simulink model "DOF4_v5"  (R2018a)
settings: Solver=VariableStepAuto  StartTime=0.0  StopTime=20  RelTol=1e-3
undefined symbols (not defined in the file or in its folder): X, Y, Z
libraries: sm_lib x20, nesl_utility x12, simulink x5
settings Model: Creator=sty  LastModifiedBy=sty

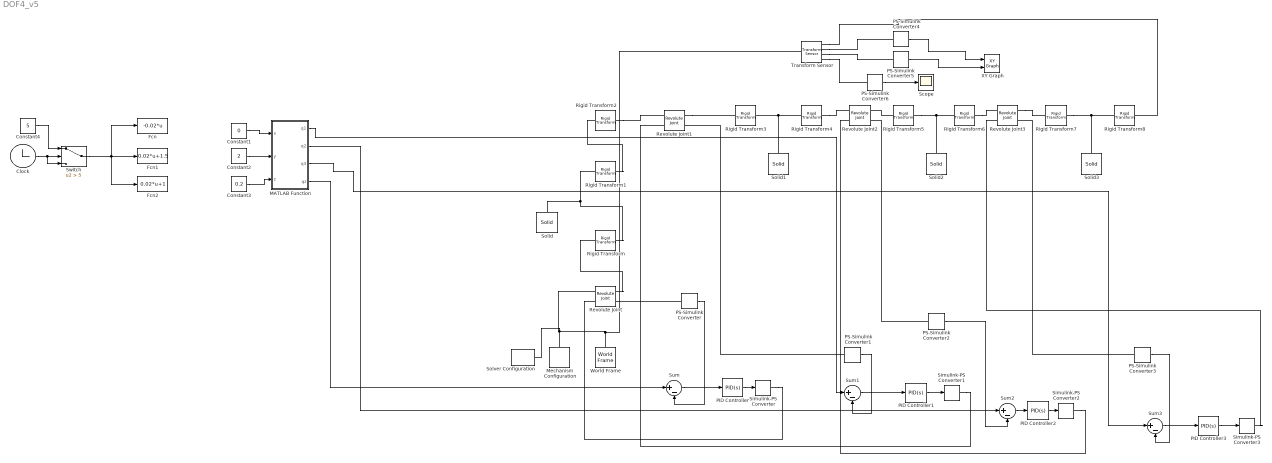
== system DOF4_v5 ==
  Clock : Clock
  Constant1 : Constant  Value=0
  Constant2 : Constant  Value=2
  Constant3 : Constant  Value=0.2
  Constant4 : Constant  Value=5
  Fcn : Fcn  Expr=-0.02*u
  Fcn1 : Fcn  Expr=0.02*u+1.5
  Fcn2 : Fcn  Expr=0.02*u+1
  MATLAB Function : MATLAB Function  TreatAsAtomicUnit=on
  Mechanism Configuration : sm_lib/Utilities/Mechanism Configuration  UniformGravity=Constant  GravityVector=[0 0 0]  GravityUnits=m/s^2  LinearizationDelta=0.001
  PID Controller{,1..3} (4 alike) : simulink/Continuous/PID Controller  Controller=PID  TimeDomain=Continuous-time  SampleTime=-1  IntegratorMethod=Forward Euler  FilterMethod=Forward Euler  Form=Parallel  UseFilter=on  ControllerParametersSource=internal  P=1000  I=40  D=60  N=100  InitialConditionSource=internal  InitialConditionForIntegrator=0  InitialConditionForFilter=0  ExternalReset=none  LimitOutput=off  UpperSaturationLimit=inf  LowerSaturationLimit=-inf  LinearizeAsGain=on  AntiWindupMode=none  Kb=1  TrackingMode=off  Kt=1  PParamMin=[]  PParamMax=[]  IParamMin=[]  IParamMax=[]  DParamMin=[]  DParamMax=[]  NParamMin=[]  NParamMax=[]  KbParamMin=[]  KbParamMax=[]  KtParamMin=[]  KtParamMax=[]  POutMin=[]  POutMax=[]  IOutMin=[]  IOutMax=[]  DOutMin=[]  DOutMax=[]  NOutMin=[]  NOutMax=[]  KbOutMin=[]  KbOutMax=[]  KtOutMin=[]  KtOutMax=[]  IntegratorOutMin=[]  IntegratorOutMax=[]  FilterOutMin=[]  FilterOutMax=[]  SumOutMin=[]  SumOutMax=[]  SumI1OutMin=[]  SumI1OutMax=[]  SumI2OutMin=[]  SumI2OutMax=[]  SumI3OutMin=[]  SumI3OutMax=[]  SumDOutMin=[]  SumDOutMax=[]  SaturationOutMin=[]  SaturationOutMax=[]  IntegratorContinuousStateAttributes=''  IntegratorStateMustResolveToSignalObject=off  IntegratorRTWStateStorageClass=Auto  FilterContinuousStateAttributes=''  FilterStateMustResolveToSignalObject=off  FilterRTWStateStorageClass=Auto  DifferentiatorICPrevScaledInput=0  DifferentiatorOutMin=[]  DifferentiatorOutMax=[]  FilterDiffOutCoefMin=[]  FilterDiffOutCoefMax=[]  SumDenOutMin=[]  SumDenOutMax=[]  SumNumOutMin=[]  SumNumOutMax=[]  ReciprocalOutMin=[]  ReciprocalOutMax=[]  DivideOutMin=[]  DivideOutMax=[]  TunerSelectOption=Transfer Function Based (PID Tuner App)
  PS-Simulink Converter{,1..6} (7 alike) : nesl_utility/PS-Simulink Converter  PhysicalDomain=network_engine_domain  SubClassName=ps_output  LeftPortType=input  RightPortType=output  PseudoPeriodic=off  Frequencies=[]  Unit=1  AffineConversion=off
  Revolute Joint{,1..3} (4 alike) : sm_lib/Joints/Revolute Joint  SenseConstraintForce=off  SenseConstraintForceX=off  SenseConstraintForceY=off  SenseConstraintForceZ=off  SenseConstraintTorque=off  SenseConstraintTorqueX=off  SenseConstraintTorqueY=off  SenseConstraintTorqueZ=off  SenseTotalForce=off  SenseTotalForceX=off  SenseTotalForceY=off  SenseTotalForceZ=off  SenseTotalTorque=off  SenseTotalTorqueX=off  SenseTotalTorqueY=off  SenseTotalTorqueZ=off  CompositeWrenchDir=FollowerOnBase  CompositeWrenchFrame=BaseFrame  EquilibriumPosition=0  EquilibriumPositionUnits=deg  SpringStiffness=0  SpringStiffnessUnits=N*m/deg  DampingCoefficient=0  DampingCoefficientUnits=N*m/(deg/s)  TorqueActuationMode=InputTorque  MotionActuationMode=ComputedMotion  SensePosition=on  SenseVelocity=off  SenseAcceleration=off  SenseTorqueForce=off  PositionTargetSpecify=off  PositionTargetPriority=High  PositionTargetValue=0  PositionTargetValueUnits=deg  VelocityTargetSpecify=off  VelocityTargetPriority=High  VelocityTargetValue=0  VelocityTargetValueUnits=deg/s
  Rigid Transform : sm_lib/Frames and Transforms/Rigid Transform  TranslationMethod=StandardAxis  TranslationStandardOffset=0.1  TranslationLengthUnit=m  TranslationStandardAxis=+Z  TranslationCartesianOffset=[0 0 0]  TranslationROffset=0  TranslationROffsetUnits=m  TranslationZOffset=0  TranslationZOffsetUnits=m  TranslationThetaOffset=0  TranslationThetaOffsetUnits=deg  RotationMethod=None  RotationAngleUnits=deg  RotationStandardAxis=+Z  RotationAngle=0.0  RotationArbitraryAxis=[0 0 1]  FollAlignAxisA=+X  BaseAlignAxisA=+Y  FollAlignAxisB=+Y  BaseAlignAxisB=+Z  RotationSequenceAxes=FollowerAxes  RotationSequence=XYX  RotationSequenceAngles=[0 0 0]  RotationSequenceAnglesUnits=deg  RotationMatrix=[1 0 0; 0 1 0; 0 0 1]
  Rigid Transform1 : sm_lib/Frames and Transforms/Rigid Transform  TranslationMethod=StandardAxis  TranslationStandardOffset=0.1  TranslationLengthUnit=m  TranslationStandardAxis=+Z  TranslationCartesianOffset=[0 0 0]  TranslationROffset=0  TranslationROffsetUnits=m  TranslationZOffset=0  TranslationZOffsetUnits=m  TranslationThetaOffset=0  TranslationThetaOffsetUnits=deg  RotationMethod=None  RotationAngleUnits=deg  RotationStandardAxis=+Z  RotationAngle=0.0  RotationArbitraryAxis=[0 0 1]  FollAlignAxisA=+X  BaseAlignAxisA=+Y  FollAlignAxisB=+Y  BaseAlignAxisB=+Z  RotationSequenceAxes=FollowerAxes  RotationSequence=XYX  RotationSequenceAngles=[0 0 0]  RotationSequenceAnglesUnits=deg  RotationMatrix=[1 0 0; 0 1 0; 0 0 1]
  Rigid Transform2 : sm_lib/Frames and Transforms/Rigid Transform  TranslationMethod=None  TranslationStandardOffset=0.1  TranslationLengthUnit=m  TranslationStandardAxis=+Z  TranslationCartesianOffset=[0 0 0]  TranslationROffset=0  TranslationROffsetUnits=m  TranslationZOffset=0  TranslationZOffsetUnits=m  TranslationThetaOffset=0  TranslationThetaOffsetUnits=deg  RotationMethod=StandardAxis  RotationAngleUnits=deg  RotationStandardAxis=+Y  RotationAngle=-90  RotationArbitraryAxis=[0 0 1]  FollAlignAxisA=+X  BaseAlignAxisA=+Y  FollAlignAxisB=+Y  BaseAlignAxisB=+Z  RotationSequenceAxes=FollowerAxes  RotationSequence=XYX  RotationSequenceAngles=[0 0 0]  RotationSequenceAnglesUnits=deg  RotationMatrix=[1 0 0; 0 1 0; 0 0 1]
  Rigid Transform{3..6} (4 alike) : sm_lib/Frames and Transforms/Rigid Transform  TranslationMethod=StandardAxis  TranslationStandardOffset=0.5  TranslationLengthUnit=m  TranslationStandardAxis=+Y  TranslationCartesianOffset=[0 0 0]  TranslationROffset=0  TranslationROffsetUnits=m  TranslationZOffset=0  TranslationZOffsetUnits=m  TranslationThetaOffset=0  TranslationThetaOffsetUnits=deg  RotationMethod=None  RotationAngleUnits=deg  RotationStandardAxis=+Z  RotationAngle=0.0  RotationArbitraryAxis=[0 0 1]  FollAlignAxisA=+X  BaseAlignAxisA=+Y  FollAlignAxisB=+Y  BaseAlignAxisB=+Z  RotationSequenceAxes=FollowerAxes  RotationSequence=XYX  RotationSequenceAngles=[0 0 0]  RotationSequenceAnglesUnits=deg  RotationMatrix=[1 0 0; 0 1 0; 0 0 1]
  Rigid Transform7 : sm_lib/Frames and Transforms/Rigid Transform  TranslationMethod=StandardAxis  TranslationStandardOffset=0.25  TranslationLengthUnit=m  TranslationStandardAxis=+Y  TranslationCartesianOffset=[0 0 0]  TranslationROffset=0  TranslationROffsetUnits=m  TranslationZOffset=0  TranslationZOffsetUnits=m  TranslationThetaOffset=0  TranslationThetaOffsetUnits=deg  RotationMethod=None  RotationAngleUnits=deg  RotationStandardAxis=+Z  RotationAngle=0.0  RotationArbitraryAxis=[0 0 1]  FollAlignAxisA=+X  BaseAlignAxisA=+Y  FollAlignAxisB=+Y  BaseAlignAxisB=+Z  RotationSequenceAxes=FollowerAxes  RotationSequence=XYX  RotationSequenceAngles=[0 0 0]  RotationSequenceAnglesUnits=deg  RotationMatrix=[1 0 0; 0 1 0; 0 0 1]
  Rigid Transform8 : sm_lib/Frames and Transforms/Rigid Transform  TranslationMethod=StandardAxis  TranslationStandardOffset=0.25  TranslationLengthUnit=m  TranslationStandardAxis=+Y  TranslationCartesianOffset=[0 0 0]  TranslationROffset=0  TranslationROffsetUnits=m  TranslationZOffset=0  TranslationZOffsetUnits=m  TranslationThetaOffset=0  TranslationThetaOffsetUnits=deg  RotationMethod=None  RotationAngleUnits=deg  RotationStandardAxis=+Z  RotationAngle=0.0  RotationArbitraryAxis=[0 0 1]  FollAlignAxisA=+X  BaseAlignAxisA=+Y  FollAlignAxisB=+Y  BaseAlignAxisB=+Z  RotationSequenceAxes=FollowerAxes  RotationSequence=XYX  RotationSequenceAngles=[0 0 0]  RotationSequenceAnglesUnits=deg  RotationMatrix=[1 0 0; 0 1 0; 0 0 1]
  Scope : Scope
  Simulink-PS Converter{,1..3} (4 alike) : nesl_utility/Simulink-PS Converter  PhysicalDomain=network_engine_domain  SubClassName=ps_input  LeftPortType=input  RightPortType=output  PseudoPeriodic=off  Frequencies=[]  NoiseDistribution=none  NoiseParameters=[]  Unit=1  AffineConversion=off  FilteringAndDerivatives=provide  SimscapeFilterOrder=1  InputFilterTimeConstant=0.001  UdotUserProvided=0
  Solid : sm_lib/Body Elements/Solid  InertiaType=CalculateFromGeometry  Mass=1  MassUnits=kg  CenterOfMass=[0 0 0]  CenterOfMassUnits=m  MomentsOfInertia=[1 1 1]  MomentsOfInertiaUnits=kg*m^2  ProductsOfInertia=[0 0 0]  ProductsOfInertiaUnits=kg*m^2  DensityBased=on  Density=1000  DensityUnits=kg/m^3  DoExposeReferenceFrame=on  SerializedFrames=<Frames/>  GraphicType=FromGeometry  MarkerShape=Sphere  MarkerSize=10  GraphicVisPropType=SimpleVisualProperties  GraphicDiffuseColor=[0.0 0.0 1.0]  GraphicSpecularColor=[0.5 0.5 0.5 1.0]  GraphicAmbientColor=[0.15 0.15 0.15 1.0]  GraphicEmissiveColor=[0.0 0.0 0.0 1.0]  GraphicShininess=75  GraphicOpacity=1.0  GeometryShape=Brick  RectangleSize=[1 1]  RectangleSizeUnits=m  BrickDimensions=[0.1 0.1 0.2]  BrickDimensionUnits=m  CylinderRadius=1  CylinderRadiusUnits=m  CylinderLength=1  CylinderLengthUnits=m  SphereRadius=1  SphereRadiusUnits=m  EllipsoidRadii=[1 1 1]  EllipsoidRadiiUnits=m  ExtrusionCrossSection=[1 1; -1 1; -1 -1; 1 -1]  ExtrusionCrossSectionUnits=m  ExtrusionLength=1  ExtrusionLengthUnits=m  PolygonNumSides=3  PolygonOuterRadius=1  PolygonOuterRadiusUnits=m  ExtGeomFileType=STEP  ExtGeomFileUnits=m  RevolutionCrossSection=[1 1; 1 -1; 2 -1; 2 1]  RevolutionCrossSectionUnits=m  RevolutionExtent=Full  RevolutionAngle=180  RevolutionAngleUnits=deg
  Solid1 : sm_lib/Body Elements/Solid  InertiaType=CalculateFromGeometry  Mass=1  MassUnits=kg  CenterOfMass=[0 0 0]  CenterOfMassUnits=m  MomentsOfInertia=[1 1 1]  MomentsOfInertiaUnits=kg*m^2  ProductsOfInertia=[0 0 0]  ProductsOfInertiaUnits=kg*m^2  DensityBased=on  Density=1000  DensityUnits=kg/m^3  DoExposeReferenceFrame=on  SerializedFrames=<Frames/>  GraphicType=FromGeometry  MarkerShape=Sphere  MarkerSize=10  GraphicVisPropType=SimpleVisualProperties  GraphicDiffuseColor=[1.0 1.0 0.2]  GraphicSpecularColor=[0.5 0.5 0.5 1.0]  GraphicAmbientColor=[0.15 0.15 0.15 1.0]  GraphicEmissiveColor=[0.0 0.0 0.0 1.0]  GraphicShininess=75  GraphicOpacity=1.0  GeometryShape=Brick  RectangleSize=[1 1]  RectangleSizeUnits=m  BrickDimensions=[0.1 1 0.1]  BrickDimensionUnits=m  CylinderRadius=1  CylinderRadiusUnits=m  CylinderLength=1  CylinderLengthUnits=m  SphereRadius=1  SphereRadiusUnits=m  EllipsoidRadii=[1 1 1]  EllipsoidRadiiUnits=m  ExtrusionCrossSection=[1 1; -1 1; -1 -1; 1 -1]  ExtrusionCrossSectionUnits=m  ExtrusionLength=1  ExtrusionLengthUnits=m  PolygonNumSides=3  PolygonOuterRadius=1  PolygonOuterRadiusUnits=m  ExtGeomFileType=STEP  ExtGeomFileUnits=m  RevolutionCrossSection=[1 1; 1 -1; 2 -1; 2 1]  RevolutionCrossSectionUnits=m  RevolutionExtent=Full  RevolutionAngle=180  RevolutionAngleUnits=deg
  Solid2 : sm_lib/Body Elements/Solid  InertiaType=CalculateFromGeometry  Mass=1  MassUnits=kg  CenterOfMass=[0 0 0]  CenterOfMassUnits=m  MomentsOfInertia=[1 1 1]  MomentsOfInertiaUnits=kg*m^2  ProductsOfInertia=[0 0 0]  ProductsOfInertiaUnits=kg*m^2  DensityBased=on  Density=1000  DensityUnits=kg/m^3  DoExposeReferenceFrame=on  SerializedFrames=<Frames/>  GraphicType=FromGeometry  MarkerShape=Sphere  MarkerSize=10  GraphicVisPropType=SimpleVisualProperties  GraphicDiffuseColor=[0.0 0.0 1.0]  GraphicSpecularColor=[0.5 0.5 0.5 1.0]  GraphicAmbientColor=[0.15 0.15 0.15 1.0]  GraphicEmissiveColor=[0.0 0.0 0.0 1.0]  GraphicShininess=75  GraphicOpacity=1.0  GeometryShape=Brick  RectangleSize=[1 1]  RectangleSizeUnits=m  BrickDimensions=[0.1 1 0.1]  BrickDimensionUnits=m  CylinderRadius=1  CylinderRadiusUnits=m  CylinderLength=1  CylinderLengthUnits=m  SphereRadius=1  SphereRadiusUnits=m  EllipsoidRadii=[1 1 1]  EllipsoidRadiiUnits=m  ExtrusionCrossSection=[1 1; -1 1; -1 -1; 1 -1]  ExtrusionCrossSectionUnits=m  ExtrusionLength=1  ExtrusionLengthUnits=m  PolygonNumSides=3  PolygonOuterRadius=1  PolygonOuterRadiusUnits=m  ExtGeomFileType=STEP  ExtGeomFileUnits=m  RevolutionCrossSection=[1 1; 1 -1; 2 -1; 2 1]  RevolutionCrossSectionUnits=m  RevolutionExtent=Full  RevolutionAngle=180  RevolutionAngleUnits=deg
  Solid3 : sm_lib/Body Elements/Solid  InertiaType=CalculateFromGeometry  Mass=1  MassUnits=kg  CenterOfMass=[0 0 0]  CenterOfMassUnits=m  MomentsOfInertia=[1 1 1]  MomentsOfInertiaUnits=kg*m^2  ProductsOfInertia=[0 0 0]  ProductsOfInertiaUnits=kg*m^2  DensityBased=on  Density=1000  DensityUnits=kg/m^3  DoExposeReferenceFrame=on  SerializedFrames=<Frames/>  GraphicType=FromGeometry  MarkerShape=Sphere  MarkerSize=10  GraphicVisPropType=SimpleVisualProperties  GraphicDiffuseColor=[1.0 0.0 0.0]  GraphicSpecularColor=[0.5 0.5 0.5 1.0]  GraphicAmbientColor=[0.15 0.15 0.15 1.0]  GraphicEmissiveColor=[0.0 0.0 0.0 1.0]  GraphicShininess=75  GraphicOpacity=1.0  GeometryShape=Brick  RectangleSize=[1 1]  RectangleSizeUnits=m  BrickDimensions=[0.1 0.5 0.1]  BrickDimensionUnits=m  CylinderRadius=1  CylinderRadiusUnits=m  CylinderLength=1  CylinderLengthUnits=m  SphereRadius=1  SphereRadiusUnits=m  EllipsoidRadii=[1 1 1]  EllipsoidRadiiUnits=m  ExtrusionCrossSection=[1 1; -1 1; -1 -1; 1 -1]  ExtrusionCrossSectionUnits=m  ExtrusionLength=1  ExtrusionLengthUnits=m  PolygonNumSides=3  PolygonOuterRadius=1  PolygonOuterRadiusUnits=m  ExtGeomFileType=STEP  ExtGeomFileUnits=m  RevolutionCrossSection=[1 1; 1 -1; 2 -1; 2 1]  RevolutionCrossSectionUnits=m  RevolutionExtent=Full  RevolutionAngle=180  RevolutionAngleUnits=deg
  Solver Configuration : nesl_utility/Solver Configuration  PhysicalDomain=network_engine_domain  SubClassName=solver  LeftPortType=input  RightPortType=generic  Tones=[]  Harmonics=[]  SimulateNoise=off  Profile=off  UseLocalSampling=off  EnableSwitchedLinearOptims=on  FrequencyDomain=off  UseCCode=off  RelTol=0.001  AbsTol=1e-06  MinStep=1e-09  ToWorkspace=off  RevertToSquareIcSolve=off  NumHomotopyIterations=100  PhasorMode=off  PhasorModeNumHarmonics=1  DoDC=off  ResidualTolerance=1e-09  UseLocalSolver=off  LocalSolverChoice=NE_BACKWARD_EULER_ADVANCER  LocalSolverSampleTime=0.001  DoFixedCost=off  MaxNonlinIter=3  MaxModeIter=2  LinearAlgebra=Sparse  EquationFormulation=NE_TIME_EF  DelaysMemoryBudget=1024  AutomaticFiltering=on  FilteringTimeConstant=0.001
  Sum{,1..3} (4 alike) : Sum  Inputs=|+-
  Switch : Switch  Criteria=u2 > Threshold  Threshold=5
  Transform Sensor : sm_lib/Frames and Transforms/Transform Sensor  MeasurementFrame=World  SenseAngle=off  SenseAxis=off  SenseAngle1=off  SenseAngle2=off  SenseAngle3=off  SenseQ=off  SenseR=off  SenseOmegaX=off  SenseOmegaY=off  SenseOmegaZ=off  SenseOmega1=off  SenseOmega2=off  SenseOmega3=off  SenseQDot=off  SenseRDot=off  SenseAlphaX=off  SenseAlphaY=off  SenseAlphaZ=off  SenseAlpha1=off  SenseAlpha2=off  SenseAlpha3=off  SenseQDDot=off  SenseRDDot=off  SenseX=on  SenseY=on  SenseZ=on  SenseRad=off  SenseAzim=off  SenseDist=off  SenseInc=off  SenseXDot=off  SenseYDot=off  SenseZDot=off  SenseRadDot=off  SenseAzimDot=off  SenseDistDot=off  SenseIncDot=off  SenseXDDot=off  SenseYDDot=off  SenseZDDot=off  SenseRadDDot=off  SenseAzimDDot=off  SenseDistDDot=off  SenseIncDDot=off
  World Frame : sm_lib/Frames and Transforms/World Frame
  XY Graph : simulink/Sinks/XY Graph  xmin=-0.5  xmax=1.5  ymin=-0.5  ymax=1.5  st=-1
  wires:
  Sum/1 -> PID Controller/1
  PID Controller/1 -> Simulink-PS Converter/1
  MATLAB Function/4(qz) -> Sum/1
  PS-Simulink Converter1/1 -> Sum1/2
  Sum1/1 -> PID Controller1/1
  PID Controller1/1 -> Simulink-PS Converter1/1
  MATLAB Function/1(q1) -> Sum1/1
  Sum2/1 -> PID Controller2/1
  PID Controller2/1 -> Simulink-PS Converter2/1
  MATLAB Function/2(q2) -> Sum2/1
  PS-Simulink Converter/1 -> Sum/2
  PS-Simulink Converter2/1 -> Sum2/2
  Sum3/1 -> PID Controller3/1
  PID Controller3/1 -> Simulink-PS Converter3/1
  MATLAB Function/3(q3) -> Sum3/1
  PS-Simulink Converter3/1 -> Sum3/2
  Switch/1 -> Fcn2/1, Fcn1/1, Fcn/1
  Clock/1 -> Switch/3, Switch/2
  Constant4/1 -> Switch/1
  Constant1/1 -> MATLAB Function/1(x)
  Constant2/1 -> MATLAB Function/2(y)
  Constant3/1 -> MATLAB Function/3(z)
  PS-Simulink Converter4/1 -> XY Graph/1
  PS-Simulink Converter5/1 -> XY Graph/2
  PS-Simulink Converter6/1 -> Scope/1
  connections:
  World Frame/RConn1 -- Transform Sensor/LConn1 -- Revolute Joint/LConn1 -- Solver Configuration/RConn1 -- Mechanism Configuration/RConn1
  Rigid Transform/RConn1 -- Solid/RConn1 -- Rigid Transform1/LConn1
  Revolute Joint/RConn1 -- Rigid Transform/LConn1
  Rigid Transform1/RConn1 -- Rigid Transform2/LConn1
  Rigid Transform2/RConn1 -- Revolute Joint1/LConn1
  Revolute Joint1/RConn1 -- Rigid Transform3/LConn1
  Rigid Transform4/LConn1 -- Solid1/RConn1 -- Rigid Transform3/RConn1
  Rigid Transform4/RConn1 -- Revolute Joint2/LConn1
  Rigid Transform5/LConn1 -- Revolute Joint2/RConn1
  Rigid Transform5/RConn1 -- Rigid Transform6/LConn1 -- Solid2/RConn1
  Rigid Transform6/RConn1 -- Revolute Joint3/LConn1
  Revolute Joint3/RConn1 -- Rigid Transform7/LConn1
  Rigid Transform7/RConn1 -- Rigid Transform8/LConn1 -- Solid3/RConn1
  Simulink-PS Converter/RConn1 -- Revolute Joint/LConn2
  PS-Simulink Converter/LConn1 -- Revolute Joint/RConn2
  Simulink-PS Converter1/RConn1 -- Revolute Joint1/LConn2
  PS-Simulink Converter1/LConn1 -- Revolute Joint1/RConn2
  Simulink-PS Converter2/RConn1 -- Revolute Joint2/LConn2
  PS-Simulink Converter2/LConn1 -- Revolute Joint2/RConn2
  PS-Simulink Converter3/LConn1 -- Revolute Joint3/RConn2
  Simulink-PS Converter3/RConn1 -- Revolute Joint3/LConn2
  Transform Sensor/RConn1 -- Rigid Transform8/RConn1
  Transform Sensor/RConn3 -- PS-Simulink Converter5/LConn1
  Transform Sensor/RConn2 -- PS-Simulink Converter4/LConn1
  Transform Sensor/RConn4 -- PS-Simulink Converter6/LConn1

== matlab function DOF4_v5/MATLAB Function ==
  data: x input; q1 output; y input; q2 output; z input; q3 output; qz output
function [q1,q2,q3,qz] = fcn(x,y,z)

Lz = 0.2;
L1 = 1;
L2 = 1;
L3 = 0.5;
theta = pi/3;

z=z+0.86;


q1 =-(2*atan((2*L1*(z - L3 * sin(theta)-Lz) - (L1^2*((- L1^2 + 2*L1*L2 - L2^2 + (sqrt(x^2+y^2) - L3*cos(theta))^2 + (z - L3 * sin(theta)-Lz)^2)*(L1^2 + 2*L1*L2 + L2^2 - (sqrt(x^2+y^2) - L3*cos(theta))^2 - (z - L3 * sin(theta)-Lz)^2))^(1/2))/(- L1^2 + 2*L1*L2 - L2^2 + (sqrt(x^2+y^2) - L3*cos(theta))^2 + (z - L3 * sin(theta)-Lz)^2) - (L2^2*((- L1^2 + 2*L1*L2 - L2^2 + (sqrt(x^2+y^2) - L3*cos(theta))^2 + (z - L3 * sin(theta)-Lz)^2)*(L1^2 + 2*L1*L2 + L2^2 - (sqrt(x^2+y^2) - L3*cos(theta))^2 - (z - L3 * sin(theta)-Lz)^2))^(1/2))/(- L1^2 + 2*L1*L2 - L2^2 + (sqrt(x^2+y^2) - L3*cos(theta))^2 + (z - L3 * sin(theta)-Lz)^2) + ((sqrt(x^2+y^2) - L3*cos(theta))^2*((- L1^2 + 2*L1*L2 - L2^2 + (sqrt(x^2+y^2) - L3*cos(theta))^2 + (z - L3 * sin(theta)-Lz)^2)*(L1^2 + 2*L1*L2 + L2^2 - (sqrt(x^2+y^2) - L3*cos(theta))^2 - (z - L3 * sin(theta)-Lz)^2))^(1/2))/(- L1^2 + 2*L1*L2 - L2^2 + (sqrt(x^2+y^2) - L3*cos(theta))^2 + (z - L3 * sin(theta)-Lz)^2) + ((z - L3 * sin(theta)-Lz)^2*((- L1^2 + 2*L1*L2 - L2^2 + (sqrt(x^2+y^2) - L3*cos(theta))^2 + (z - L3 * sin(theta)-Lz)^2)*(L1^2 + 2*L1*L2 + L2^2 - (sqrt(x^2+y^2) - L3*cos(theta))^2 - (z - L3 * sin(theta)-Lz)^2))^(1/2))/(- L1^2 + 2*L1*L2 - L2^2 + (sqrt(x^2+y^2) - L3*cos(theta))^2 + (z - L3 * sin(theta)-Lz)^2) + (2*L1*L2*((- L1^2 + 2*L1*L2 - L2^2 + (sqrt(x^2+y^2) - L3*cos(theta))^2 + (z - L3 * sin(theta)-Lz)^2)*(L1^2 + 2*L1*L2 + L2^2 - (sqrt(x^2+y^2) - L3*cos(theta))^2 - (z - L3 * sin(theta)-Lz)^2))^(1/2))/(- L1^2 + 2*L1*L2 - L2^2 + (sqrt(x^2+y^2) - L3*cos(theta))^2 + (z - L3 * sin(theta)-Lz)^2))/(L1^2 + 2*L1*(sqrt(x^2+y^2) - L3*cos(theta)) - L2^2 + (sqrt(x^2+y^2) - L3*cos(theta))^2 + (z - L3 * sin(theta)-Lz)^2)));
 
 %2*atan((2*L1*(z - L3 * sin(theta)-Lz) - (L1^2*((- L1^2 + 2*L1*L2 - L2^2 + (sqrt(x^2+y^2) - L3*cos(theta))^2 + (z - L3 * sin(theta)-Lz)^2)*(L1^2 + 2*L1*L2 + L2^2 - (sqrt(x^2+y^2) - L3*cos(theta))^2 - (z - L3 * sin(theta)-Lz)^2))^(1/2))/(- L1^2 + 2*L1*L2 - L2^2 + (sqrt(x^2+y^2) - L3*cos(theta))^2 + (z - L3 * sin(theta)-Lz)^2) - (L2^2*((- L1^2 + 2*L1*L2 - L2^2 + (sqrt(x^2+y^2) - L3*cos(theta))^2 + (z - L3 * sin(theta)-Lz)^2)*(L1^2 + 2*L1*L2 + L2^2 - (sqrt(x^2+y^2) - L3*cos(theta))^2 - (z - L3 * sin(theta)-Lz)^2))^(1/2))/(- L1^2 + 2*L1*L2 - L2^2 + (sqrt(x^2+y^2) - L3*cos(theta))^2 + (z - L3 * sin(theta)-Lz)^2) + ((sqrt(x^2+y^2) - L3*cos(theta))^2*((- L1^2 + 2*L1*L2 - L2^2 + (sqrt(x^2+y^2) - L3*cos(theta))^2 + (z - L3 * sin(theta)-Lz)^2)*(L1^2 + 2*L1*L2 + L2^2 - (sqrt(x^2+y^2) - L3*cos(theta))^2 - (z - L3 * sin(theta)-Lz)^2))^(1/2))/(- L1^2 + 2*L1*L2 - L2^2 + (sqrt(x^2+y^2) - L3*cos(theta))^2 + (z - L3 * sin(theta)-Lz)^2) + ((z - L3 * sin(theta)-Lz)^2*((- L1^2 + 2*L1*L2 - L2^2 + (sqrt(x^2+y^2) - L3*cos(theta))^2 + (z - L3 * sin(theta)-Lz)^2)*(L1^2 + 2*L1*L2 + L2^2 - (sqrt(x^2+y^2) - L3*cos(theta))^2 - (z - L3 * sin(theta)-Lz)^2))^(1/2))/(- L1^2 + 2*L1*L2 - L2^2 + (sqrt(x^2+y^2) - L3*cos(theta))^2 + (z - L3 * sin(theta)-Lz)^2) + (2*L1*L2*((- L1^2 + 2*L1*L2 - L2^2 + (sqrt(x^2+y^2) - L3*cos(theta))^2 + (z - L3 * sin(theta)-Lz)^2)*(L1^2 + 2*L1*L2 + L2^2 - (sqrt(x^2+y^2) - L3*cos(theta))^2 - (z - L3 * sin(theta)-Lz)^2))^(1/2))/(- L1^2 + 2*L1*L2 - L2^2 + (sqrt(x^2+y^2) - L3*cos(theta))^2 + (z - L3 * sin(theta)-Lz)^2))/(L1^2 + 2*L1*(sqrt(x^2+y^2) - L3*cos(theta)) - L2^2 + (sqrt(x^2+y^2) - L3*cos(theta))^2 + (z - L3 * sin(theta)-Lz)^2))
 %2*atan((2*L1*(z - L3 * sin(theta)-Lz) + (L1^2*((- L1^2 + 2*L1*L2 - L2^2 + (sqrt(x^2+y^2) - L3*cos(theta))^2 + (z - L3 * sin(theta)-Lz)^2)*(L1^2 + 2*L1*L2 + L2^2 - (sqrt(x^2+y^2) - L3*cos(theta))^2 - (z - L3 * sin(theta)-Lz)^2))^(1/2))/(- L1^2 + 2*L1*L2 - L2^2 + (sqrt(x^2+y^2) - L3*cos(theta))^2 + (z - L3 * sin(theta)-Lz)^2) + (L2^2*((- L1^2 + 2*L1*L2 - L2^2 + (sqrt(x^2+y^2) - L3*cos(theta))^2 + (z - L3 * sin(theta)-Lz)^2)*(L1^2 + 2*L1*L2 + L2^2 - (sqrt(x^2+y^2) - L3*cos(theta))^2 - (z - L3 * sin(theta)-Lz)^2))^(1/2))/(- L1^2 + 2*L1*L2 - L2^2 + (sqrt(x^2+y^2) - L3*cos(theta))^2 + (z - L3 * sin(theta)-Lz)^2) - ((sqrt(x^2+y^2) - L3*cos(theta))^2*((- L1^2 + 2*L1*L2 - L2^2 + (sqrt(x^2+y^2) - L3*cos(theta))^2 + (z - L3 * sin(theta)-Lz)^2)*(L1^2 + 2*L1*L2 + L2^2 - (sqrt(x^2+y^2) - L3*cos(theta))^2 - (z - L3 * sin(theta)-Lz)^2))^(1/2))/(- L1^2 + 2*L1*L2 - L2^2 + (sqrt(x^2+y^2) - L3*cos(theta))^2 + (z - L3 * sin(theta)-Lz)^2) - ((z - L3 * sin(theta)-Lz)^2*((- L1^2 + 2*L1*L2 - L2^2 + (sqrt(x^2+y^2) - L3*cos(theta))^2 + (z - L3 * sin(theta)-Lz)^2)*(L1^2 + 2*L1*L2 + L2^2 - (sqrt(x^2+y^2) - L3*cos(theta))^2 - (z - L3 * sin(theta)-Lz)^2))^(1/2))/(- L1^2 + 2*L1*L2 - L2^2 + (sqrt(x^2+y^2) - L3*cos(theta))^2 + (z - L3 * sin(theta)-Lz)^2) - (2*L1*L2*((- L1^2 + 2*L1*L2 - L2^2 + (sqrt(x^2+y^2) - L3*cos(theta))^2 + (z - L3 * sin(theta)-Lz)^2)*(L1^2 + 2*L1*L2 + L2^2 - (sqrt(x^2+y^2) - L3*cos(theta))^2 - (z - L3 * sin(theta)-Lz)^2))^(1/2))/(- L1^2 + 2*L1*L2 - L2^2 + (sqrt(x^2+y^2) - L3*cos(theta))^2 + (z - L3 * sin(theta)-Lz)^2))/(L1^2 + 2*L1*(sqrt(x^2+y^2) - L3*cos(theta)) - L2^2 + (sqrt(x^2+y^2) - L3*cos(theta))^2 + (z - L3 * sin(theta)-Lz)^2))
 
 
q2 =-(-2*atan(((- L1^2 + 2*L1*L2 - L2^2 + (sqrt(x^2+y^2) - L3*cos(theta))^2 + (z - L3 * sin(theta)-Lz)^2)*(L1^2 + 2*L1*L2 + L2^2 - (sqrt(x^2+y^2) - L3*cos(theta))^2 - (z - L3 * sin(theta)-Lz)^2))^(1/2)/(- L1^2 + 2*L1*L2 - L2^2 + (sqrt(x^2+y^2) - L3*cos(theta))^2 + (z - L3 * sin(theta)-Lz)^2)));
 
 %-2*atan(((- L1^2 + 2*L1*L2 - L2^2 + (sqrt(x^2+y^2) - L3*cos(theta))^2 + (z - L3 * sin(theta)-Lz)^2)*(L1^2 + 2*L1*L2 + L2^2 - (sqrt(x^2+y^2) - L3*cos(theta))^2 - (z - L3 * sin(theta)-Lz)^2))^(1/2)/(- L1^2 + 2*L1*L2 - L2^2 + (sqrt(x^2+y^2) - L3*cos(theta))^2 + (z - L3 * sin(theta)-Lz)^2))
 % 2*atan(((- L1^2 + 2*L1*L2 - L2^2 + (sqrt(x^2+y^2) - L3*cos(theta))^2 + (z - L3 * sin(theta)-Lz)^2)*(L1^2 + 2*L1*L2 + L2^2 - (sqrt(x^2+y^2) - L3*cos(theta))^2 - (z - L3 * sin(theta)-Lz)^2))^(1/2)/(- L1^2 + 2*L1*L2 - L2^2 + (sqrt(x^2+y^2) - L3*cos(theta))^2 + (z - L3 * sin(theta)-Lz)^2))
  
  
q3 = theta - q1 - q2 ;


qz = -atan2(x,y);
end
